simulink model "DCMotorCLDCDC"  (R2018b)
settings: Solver=VariableStepAuto  StartTime=0.0  StopTime=10  RelTol=1e-3  EnableMultiTasking=on
InitFcn:
  | Vf=300;
libraries: powerlib x17, simulink x6, powerlib_meascontrol x2
settings Model: Creator=alireza  LastModifiedBy=Koosha
settings OptimizationCC: LifeSpan=inf
settings DebuggingCC: SFUnexpectedBacktrackingDiag=warning  SFNoUnconditionalDefaultTransitionDiag=warning
settings SFSimCC: SimUseLocalCustomCode=off
settings RTWCC: RTWUseLocalCustomCode=off
settings CodeAppCC: StateflowObjectComments=on
settings GRTTargetCC: TargetLangStandard=C89/C90 (ANSI)
settings ConfigComp: CovMetricSettings=dw  CovSaveCumulativeToWorkspaceVar=on  CovSaveSingleToWorkspaceVar=on  CovExternalEMLEnable=off
settings SimscapeCC: SimscapeNormalizeSystem=off

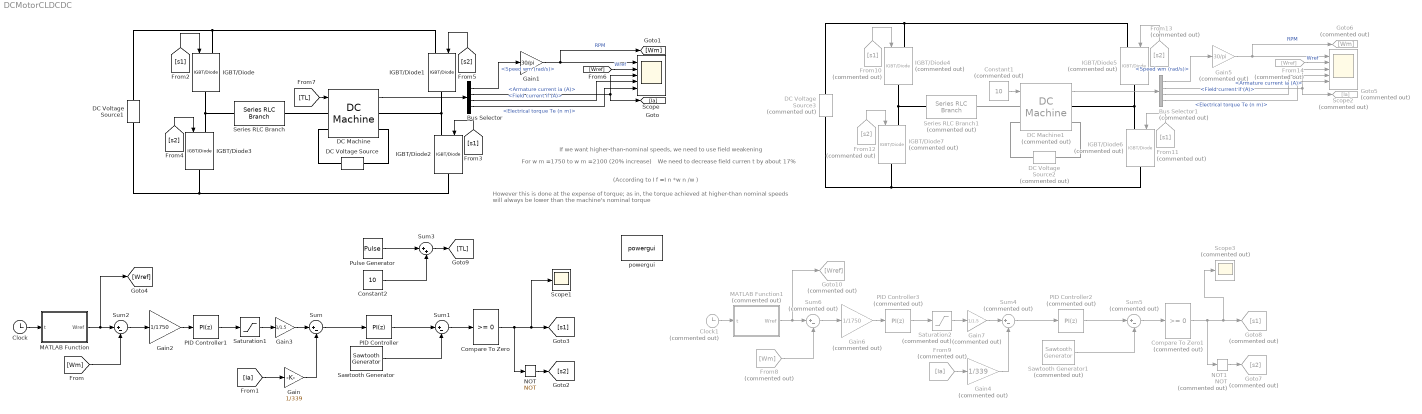
== system DCMotorCLDCDC ==
  note: We need to decrease field curren t by about 17%
  note: However this is done at the expense of torque;
      | as in, the torque achieved at higher-than nominal speeds will always be lower than the machine's nominal torque
  note: For w m =1750 to w m =2100 (20% increase)
  note: (According to I f =I n *w n /w )
  note: If we want higher-than-nominal speeds, we need to use field weakening
  Bus Selector : BusSelector  OutputSignals=Speed wm (rad/s),Armature current ia (A),Field current if (A),Electrical torque Te (n m)
  Bus Selector1 : BusSelector  Commented=on  OutputSignals=Speed wm (rad/s),Armature current ia (A),Field current if (A),Electrical torque Te (n m)
  Clock : Clock
  Clock1 : Clock  Commented=on
  Compare To Zero : simulink/Logic and Bit Operations/Compare To Zero  relop=>=  OutDataTypeStr=boolean
  Compare To Zero1 : simulink/Logic and Bit Operations/Compare To Zero  Commented=on  relop=>=  OutDataTypeStr=boolean
  Constant1 : Constant  Commented=on  Value=10
  Constant2 : Constant  Value=10
  DC Machine : powerlib/Machines/DC Machine  PresetModel=03: 5HP 500V 1750RPM Field:300V  MechanicalLoad=Torque TL  FieldType=Wound  ShowDetailedParameters=on  MeasurementBus=off  RLa=[11.2 0.1215]  RLf=[281.3 156]  Laf=1.976  MachineConstant=Torque constant (N.m/A)  Ke=1.8  Kt=1.8  J=0.02215  Bm=0.002953  Tf=0.5161  w0=0  Ifinit=1  TsPowergui=0  TsBlock=-1
  DC Machine1 : powerlib/Machines/DC Machine  Commented=on  PresetModel=03: 5HP 500V 1750RPM Field:300V  MechanicalLoad=Torque TL  FieldType=Wound  ShowDetailedParameters=on  MeasurementBus=off  RLa=[11.2 0.1215]  RLf=[281.3 156]  Laf=1.976  MachineConstant=Torque constant (N.m/A)  Ke=1.8  Kt=1.8  J=0.02215  Bm=0.002953  Tf=0.5161  w0=0  Ifinit=1  TsPowergui=0  TsBlock=-1
  DC Voltage Source : powerlib/Electrical Sources/DC Voltage Source  Amplitude=300  Measurements=None
  DC Voltage Source1 : powerlib/Electrical Sources/DC Voltage Source  Amplitude=560  Measurements=None
  DC Voltage Source2 : powerlib/Electrical Sources/DC Voltage Source  Commented=on  Amplitude=Vf  Measurements=None
  DC Voltage Source3 : powerlib/Electrical Sources/DC Voltage Source  Commented=on  Amplitude=560  Measurements=None
  From10 : From  Commented=on  GotoTag=s1
  From11 : From  Commented=on  GotoTag=s1
  From12 : From  Commented=on  GotoTag=s2
  From13 : From  Commented=on  GotoTag=s2
  From14 : From  Commented=on  GotoTag=Wref
  From8 : From  Commented=on  GotoTag=Wm
  From9 : From  Commented=on  GotoTag=Ia
  Gain : Gain  Gain=1/339
  Gain1 : Gain  Gain=30/pi
  Gain2 : Gain  Gain=1/1750
  Gain3 : Gain  Gain=1/1.5
  Gain4 : Gain  Commented=on  Gain=1/339
  Gain5 : Gain  Commented=on  Gain=30/pi
  Gain6 : Gain  Commented=on  Gain=1/1750
  Gain7 : Gain  Commented=on  Gain=1/1.5
  Goto10 : Goto  Commented=on  GotoTag=Wref
  Goto5 : Goto  Commented=on  GotoTag=Ia
  Goto6 : Goto  Commented=on  GotoTag=Wm
  Goto7 : Goto  Commented=on  GotoTag=s2
  Goto8 : Goto  Commented=on  GotoTag=s1
  IGBT/Diode{,1..3} (4 alike) : powerlib/Power Electronics/IGBT//Diode  Ron=1e-3  Rs=10e3  Cs=inf  Measurements=off
  IGBT/Diode{4..7} (4 alike) : powerlib/Power Electronics/IGBT//Diode  Commented=on  Ron=1e-3  Rs=10e3  Cs=inf  Measurements=off
  MATLAB Function : MATLAB Function  TreatAsAtomicUnit=on
  MATLAB Function1 : MATLAB Function  Commented=on  TreatAsAtomicUnit=on
  NOT : Logic  Operator=NOT  IconShape=distinctive  AllPortsSameDT=off  OutDataTypeStr=boolean
  NOT1 : Logic  Commented=on  Operator=NOT  IconShape=distinctive  AllPortsSameDT=off  OutDataTypeStr=boolean
  PID Controller : simulink/Continuous/PID Controller  Controller=PI  Form=Parallel  TimeDomain=Discrete-time  SampleTime=-1  IntegratorMethod=Forward Euler  FilterMethod=Forward Euler  ControllerParametersSource=internal  P=5  I=6  D=0  UseFilter=on  N=100  TunerSelectOption=Transfer Function Based (PID Tuner App)  InitialConditionSource=internal  InitialConditionForIntegrator=0  InitialConditionForFilter=0  DifferentiatorICPrevScaledInput=0  ExternalReset=none  TrackingMode=off  Kt=1  LimitOutput=off  UpperSaturationLimit=inf  LowerSaturationLimit=-inf  LinearizeAsGain=on  AntiWindupMode=none  Kb=1  POutMin=[]  POutMax=[]  IOutMin=[]  IOutMax=[]  DOutMin=[]  DOutMax=[]  NOutMin=[]  NOutMax=[]  SumOutMin=[]  SumOutMax=[]  SaturationOutMin=[]  SaturationOutMax=[]  PParamMin=[]  PParamMax=[]  IParamMin=[]  IParamMax=[]  DParamMin=[]  DParamMax=[]  NParamMin=[]  NParamMax=[]  KbParamMin=[]  KbParamMax=[]  KtParamMin=[]  KtParamMax=[]  KbOutMin=[]  KbOutMax=[]  KtOutMin=[]  KtOutMax=[]  IntegratorOutMin=[]  IntegratorOutMax=[]  FilterOutMin=[]  FilterOutMax=[]  SumI1OutMin=[]  SumI1OutMax=[]  SumI2OutMin=[]  SumI2OutMax=[]  SumI3OutMin=[]  SumI3OutMax=[]  SumI4OutMin=[]  SumI4OutMax=[]  SumDOutMin=[]  SumDOutMax=[]  DifferentiatorOutMin=[]  DifferentiatorOutMax=[]  FilterDiffOutCoefMin=[]  FilterDiffOutCoefMax=[]  ReciprocalOutMin=[]  ReciprocalOutMax=[]  SumDenOutMin=[]  SumDenOutMax=[]  SumNumOutMin=[]  SumNumOutMax=[]  DivideOutMin=[]  DivideOutMax=[]  IntegratorContinuousStateAttributes=''  IntegratorStateMustResolveToSignalObject=off  IntegratorRTWStateStorageClass=Auto  FilterContinuousStateAttributes=''  FilterStateMustResolveToSignalObject=off  FilterRTWStateStorageClass=Auto  ParallelPVariant=InternalParameters  IdealPVariant=Disabled  IVariant=InternalParameters  DVariant=Disabled  IntegratorVariant=Discrete  SatVariant=Disabled  AWVariant=Passthrough  PCopyVariant=Disabled  TRVariant=Disabled  FdbkBlocksVariant=Forward  IdealPFdbkVariant=Disabled  SatFdbkVariant=Disabled  DerivativeFilterVariant=Disabled  NVariant=Disabled  NCopyVariant=Disabled_SignalSpec  FilterICVariant=Disabled  IntegratorICVariant=InternalICs  ExternalResetVariant=Disabled  TRSumVariant=Passthrough  SumFdbkVariant=Disabled  SumVariant=Sum_PI
  PID Controller1 : simulink/Continuous/PID Controller  Controller=PI  Form=Parallel  TimeDomain=Discrete-time  SampleTime=-1  IntegratorMethod=Forward Euler  FilterMethod=Forward Euler  ControllerParametersSource=internal  P=10  I=10  D=0  UseFilter=on  N=100  TunerSelectOption=Transfer Function Based (PID Tuner App)  InitialConditionSource=internal  InitialConditionForIntegrator=0  InitialConditionForFilter=0  DifferentiatorICPrevScaledInput=0  ExternalReset=none  TrackingMode=off  Kt=1  LimitOutput=off  UpperSaturationLimit=inf  LowerSaturationLimit=-inf  LinearizeAsGain=on  AntiWindupMode=none  Kb=1  POutMin=[]  POutMax=[]  IOutMin=[]  IOutMax=[]  DOutMin=[]  DOutMax=[]  NOutMin=[]  NOutMax=[]  SumOutMin=[]  SumOutMax=[]  SaturationOutMin=[]  SaturationOutMax=[]  PParamMin=[]  PParamMax=[]  IParamMin=[]  IParamMax=[]  DParamMin=[]  DParamMax=[]  NParamMin=[]  NParamMax=[]  KbParamMin=[]  KbParamMax=[]  KtParamMin=[]  KtParamMax=[]  KbOutMin=[]  KbOutMax=[]  KtOutMin=[]  KtOutMax=[]  IntegratorOutMin=[]  IntegratorOutMax=[]  FilterOutMin=[]  FilterOutMax=[]  SumI1OutMin=[]  SumI1OutMax=[]  SumI2OutMin=[]  SumI2OutMax=[]  SumI3OutMin=[]  SumI3OutMax=[]  SumI4OutMin=[]  SumI4OutMax=[]  SumDOutMin=[]  SumDOutMax=[]  DifferentiatorOutMin=[]  DifferentiatorOutMax=[]  FilterDiffOutCoefMin=[]  FilterDiffOutCoefMax=[]  ReciprocalOutMin=[]  ReciprocalOutMax=[]  SumDenOutMin=[]  SumDenOutMax=[]  SumNumOutMin=[]  SumNumOutMax=[]  DivideOutMin=[]  DivideOutMax=[]  IntegratorContinuousStateAttributes=''  IntegratorStateMustResolveToSignalObject=off  IntegratorRTWStateStorageClass=Auto  FilterContinuousStateAttributes=''  FilterStateMustResolveToSignalObject=off  FilterRTWStateStorageClass=Auto  ParallelPVariant=InternalParameters  IdealPVariant=Disabled  IVariant=InternalParameters  DVariant=Disabled  IntegratorVariant=Discrete  SatVariant=Disabled  AWVariant=Passthrough  PCopyVariant=Disabled  TRVariant=Disabled  FdbkBlocksVariant=Forward  IdealPFdbkVariant=Disabled  SatFdbkVariant=Disabled  DerivativeFilterVariant=Disabled  NVariant=Disabled  NCopyVariant=Disabled_SignalSpec  FilterICVariant=Disabled  IntegratorICVariant=InternalICs  ExternalResetVariant=Disabled  TRSumVariant=Passthrough  SumFdbkVariant=Disabled  SumVariant=Sum_PI
  PID Controller2 : simulink/Continuous/PID Controller  Commented=on  Controller=PI  Form=Parallel  TimeDomain=Discrete-time  SampleTime=-1  IntegratorMethod=Forward Euler  FilterMethod=Forward Euler  ControllerParametersSource=internal  P=5  I=6  D=0  UseFilter=on  N=100  TunerSelectOption=Transfer Function Based (PID Tuner App)  InitialConditionSource=internal  InitialConditionForIntegrator=0  InitialConditionForFilter=0  DifferentiatorICPrevScaledInput=0  ExternalReset=none  TrackingMode=off  Kt=1  LimitOutput=off  UpperSaturationLimit=inf  LowerSaturationLimit=-inf  LinearizeAsGain=on  AntiWindupMode=none  Kb=1  POutMin=[]  POutMax=[]  IOutMin=[]  IOutMax=[]  DOutMin=[]  DOutMax=[]  NOutMin=[]  NOutMax=[]  SumOutMin=[]  SumOutMax=[]  SaturationOutMin=[]  SaturationOutMax=[]  PParamMin=[]  PParamMax=[]  IParamMin=[]  IParamMax=[]  DParamMin=[]  DParamMax=[]  NParamMin=[]  NParamMax=[]  KbParamMin=[]  KbParamMax=[]  KtParamMin=[]  KtParamMax=[]  KbOutMin=[]  KbOutMax=[]  KtOutMin=[]  KtOutMax=[]  IntegratorOutMin=[]  IntegratorOutMax=[]  FilterOutMin=[]  FilterOutMax=[]  SumI1OutMin=[]  SumI1OutMax=[]  SumI2OutMin=[]  SumI2OutMax=[]  SumI3OutMin=[]  SumI3OutMax=[]  SumI4OutMin=[]  SumI4OutMax=[]  SumDOutMin=[]  SumDOutMax=[]  DifferentiatorOutMin=[]  DifferentiatorOutMax=[]  FilterDiffOutCoefMin=[]  FilterDiffOutCoefMax=[]  ReciprocalOutMin=[]  ReciprocalOutMax=[]  SumDenOutMin=[]  SumDenOutMax=[]  SumNumOutMin=[]  SumNumOutMax=[]  DivideOutMin=[]  DivideOutMax=[]  IntegratorContinuousStateAttributes=''  IntegratorStateMustResolveToSignalObject=off  IntegratorRTWStateStorageClass=Auto  FilterContinuousStateAttributes=''  FilterStateMustResolveToSignalObject=off  FilterRTWStateStorageClass=Auto  ParallelPVariant=InternalParameters  IdealPVariant=Disabled  IVariant=InternalParameters  DVariant=Disabled  IntegratorVariant=Discrete  SatVariant=Disabled  AWVariant=Passthrough  PCopyVariant=Disabled  TRVariant=Disabled  FdbkBlocksVariant=Forward  IdealPFdbkVariant=Disabled  SatFdbkVariant=Disabled  DerivativeFilterVariant=Disabled  NVariant=Disabled  NCopyVariant=Disabled_SignalSpec  FilterICVariant=Disabled  IntegratorICVariant=InternalICs  ExternalResetVariant=Disabled  TRSumVariant=Passthrough  SumFdbkVariant=Disabled  SumVariant=Sum_PI
  PID Controller3 : simulink/Continuous/PID Controller  Commented=on  Controller=PI  Form=Parallel  TimeDomain=Discrete-time  SampleTime=-1  IntegratorMethod=Forward Euler  FilterMethod=Forward Euler  ControllerParametersSource=internal  P=10  I=10  D=0  UseFilter=on  N=100  TunerSelectOption=Transfer Function Based (PID Tuner App)  InitialConditionSource=internal  InitialConditionForIntegrator=0  InitialConditionForFilter=0  DifferentiatorICPrevScaledInput=0  ExternalReset=none  TrackingMode=off  Kt=1  LimitOutput=off  UpperSaturationLimit=inf  LowerSaturationLimit=-inf  LinearizeAsGain=on  AntiWindupMode=none  Kb=1  POutMin=[]  POutMax=[]  IOutMin=[]  IOutMax=[]  DOutMin=[]  DOutMax=[]  NOutMin=[]  NOutMax=[]  SumOutMin=[]  SumOutMax=[]  SaturationOutMin=[]  SaturationOutMax=[]  PParamMin=[]  PParamMax=[]  IParamMin=[]  IParamMax=[]  DParamMin=[]  DParamMax=[]  NParamMin=[]  NParamMax=[]  KbParamMin=[]  KbParamMax=[]  KtParamMin=[]  KtParamMax=[]  KbOutMin=[]  KbOutMax=[]  KtOutMin=[]  KtOutMax=[]  IntegratorOutMin=[]  IntegratorOutMax=[]  FilterOutMin=[]  FilterOutMax=[]  SumI1OutMin=[]  SumI1OutMax=[]  SumI2OutMin=[]  SumI2OutMax=[]  SumI3OutMin=[]  SumI3OutMax=[]  SumI4OutMin=[]  SumI4OutMax=[]  SumDOutMin=[]  SumDOutMax=[]  DifferentiatorOutMin=[]  DifferentiatorOutMax=[]  FilterDiffOutCoefMin=[]  FilterDiffOutCoefMax=[]  ReciprocalOutMin=[]  ReciprocalOutMax=[]  SumDenOutMin=[]  SumDenOutMax=[]  SumNumOutMin=[]  SumNumOutMax=[]  DivideOutMin=[]  DivideOutMax=[]  IntegratorContinuousStateAttributes=''  IntegratorStateMustResolveToSignalObject=off  IntegratorRTWStateStorageClass=Auto  FilterContinuousStateAttributes=''  FilterStateMustResolveToSignalObject=off  FilterRTWStateStorageClass=Auto  ParallelPVariant=InternalParameters  IdealPVariant=Disabled  IVariant=InternalParameters  DVariant=Disabled  IntegratorVariant=Discrete  SatVariant=Disabled  AWVariant=Passthrough  PCopyVariant=Disabled  TRVariant=Disabled  FdbkBlocksVariant=Forward  IdealPFdbkVariant=Disabled  SatFdbkVariant=Disabled  DerivativeFilterVariant=Disabled  NVariant=Disabled  NCopyVariant=Disabled_SignalSpec  FilterICVariant=Disabled  IntegratorICVariant=InternalICs  ExternalResetVariant=Disabled  TRSumVariant=Passthrough  SumFdbkVariant=Disabled  SumVariant=Sum_PI
  Pulse Generator : DiscretePulseGenerator  PulseType=Time based  Amplitude=10  Period=10  PulseWidth=40  PhaseDelay=4
  Saturation1 : Saturate  UpperLimit=1.5  LowerLimit=-1.5
  Saturation2 : Saturate  Commented=on  UpperLimit=1.5  LowerLimit=-1.5
  Sawtooth Generator : powerlib_meascontrol/Pulse & Signal Generators/Sawtooth Generator  Freq=5e3  Phase=90  Ts=20e-6
      settings: SourceProductName=Simscape Power Systems
  Sawtooth Generator1 : powerlib_meascontrol/Pulse & Signal Generators/Sawtooth Generator  Commented=on  Freq=5e3  Phase=90  Ts=20e-6
      settings: SourceProductName=Simscape Power Systems
  Scope : Scope  NumInputPorts=5
  Scope1 : Scope
  Scope2 : Scope  Commented=on  NumInputPorts=5
  Scope3 : Scope  Commented=on
  Series RLC Branch : powerlib/Elements/Series RLC Branch  LConnTagsString=__new0  RConnTagsString=__new0  BranchType=L  Resistance=1  Inductance=1e-3  SetiL0=off  InitialCurrent=0  Capacitance=1e-6  Setx0=off  InitialVoltage=0  Measurements=None
  Series RLC Branch1 : powerlib/Elements/Series RLC Branch  Commented=on  LConnTagsString=__new0  RConnTagsString=__new0  BranchType=L  Resistance=1  Inductance=1e-3  SetiL0=off  InitialCurrent=0  Capacitance=1e-6  Setx0=off  InitialVoltage=0  Measurements=None
  Sum : Sum  Inputs=|+-
  Sum1 : Sum  Inputs=|+-
  Sum2 : Sum  Inputs=|+-
  Sum3 : Sum  Inputs=|++
  Sum4 : Sum  Commented=on  Inputs=|+-
  Sum5 : Sum  Commented=on  Inputs=|+-
  Sum6 : Sum  Commented=on  Inputs=|+-
  powergui : powerlib/powergui  Priority=1  SimulationMode=Discrete  SampleTime=50e-6  frequency=60  Iterations=50  frequencyindice=0  Pbase=100e6  ErrMax=1e-4  UnitsV=kV  UnitsW=MW  buscounter=0  FunctionMessages=off  echomessages=off  EnableUseOfTLC=off  CurrentSourceSwitches=off  DisableSnubberDevices=off  DisableRonSwitches=off  DisableVfSwitches=off  DisplayEquations=off  SolverType=Tustin/Backward Euler (TBE)  Interpol=off  ExternalGateDelay=off  methode=off  Ts=100  x0status=blocks  SPID=off  SwTol=0  HookPort=off  RestoreLinks=warning  ResistiveCurrentMeasurement=off  Frange=[0:2:500]  Ylog=off  Xlog=on  ShowGrid=off  save=off  variable=ZData  structure=0  ZoomFFT=off  StartTime=0.0  cycles=1  DisplayStyle=1  fundamental=60  FreqAxis=off  MaxFrequency=1000  frequencyindicesteady=1  RmsSteady=1  display=off
  wires:
  Sum/1 -> PID Controller/1
  Sawtooth Generator/1 -> Sum1/2
  Sum1/1 -> Compare To Zero/1
  Clock/1 -> MATLAB Function/1(t)
  DC Machine/1 -> Bus Selector/1
  Bus Selector/1 -> Gain1/1  "<Speed wm (rad/s)>"
  MATLAB Function/1(Wref) -> [Wref], Sum2/1
  [Wm] -> Sum2/2
  Gain1/1 -> [Wm], Scope/1  "RPM"
  PID Controller1/1 -> Saturation1/1
  Compare To Zero/1 -> NOT/1, Scope1/1, [s1]
  NOT/1 -> [s2]
  [s1] -> IGBT/Diode/1
  [s1] -> IGBT/Diode2/1
  [s2] -> IGBT/Diode3/1
  [s2] -> IGBT/Diode1/1
  PID Controller/1 -> Sum1/1
  [Wref] -> Scope/2  "Wref"
  Bus Selector/2 -> [Ia], Scope/3  "<Armature current ia (A)>"
  Bus Selector/4 -> Scope/5  "<Electrical torque Te (n m)>"
  Bus Selector/3 -> Scope/4  "<Field current if (A)>"
  Saturation1/1 -> Gain3/1
  [Ia] -> Gain/1
  Gain/1 -> Sum/2
  Gain3/1 -> Sum/1
  Gain2/1 -> PID Controller1/1
  Sum2/1 -> Gain2/1
  Constant2/1 -> Sum3/2
  Sum3/1 -> [TL]
  Pulse Generator/1 -> Sum3/1
  [TL] -> DC Machine/1
  Constant1/1 -> DC Machine1/1
  Gain5/1 -> Goto6/1, Scope2/1  "RPM"
  Sum6/1 -> Gain6/1
  Gain7/1 -> Sum4/1
  Bus Selector1/4 -> Scope2/5  "<Electrical torque Te (n m)>"
  Sawtooth Generator1/1 -> Sum5/2
  PID Controller2/1 -> Sum5/1
  Gain6/1 -> PID Controller3/1
  Bus Selector1/1 -> Gain5/1  "<Speed wm (rad/s)>"
  From10/1 -> IGBT/Diode4/1
  DC Machine1/1 -> Bus Selector1/1
  From12/1 -> IGBT/Diode7/1
  From13/1 -> IGBT/Diode5/1
  From11/1 -> IGBT/Diode6/1
  NOT1/1 -> Goto7/1
  MATLAB Function1/1(Wref) -> Goto10/1, Sum6/1
  Bus Selector1/3 -> Scope2/4  "<Field current if (A)>"
  Saturation2/1 -> Gain7/1
  Bus Selector1/2 -> Goto5/1, Scope2/3  "<Armature current ia (A)>"
  Clock1/1 -> MATLAB Function1/1(t)
  From14/1 -> Scope2/2  "Wref"
  Sum4/1 -> PID Controller2/1
  Compare To Zero1/1 -> NOT1/1, Scope3/1, Goto8/1
  Sum5/1 -> Compare To Zero1/1
  PID Controller3/1 -> Saturation2/1
  From8/1 -> Sum6/2
  From9/1 -> Gain4/1
  Gain4/1 -> Sum4/2
  connections:
  IGBT/Diode1/RConn1 -- DC Machine/RConn1 -- IGBT/Diode2/LConn1
  DC Voltage Source/RConn1 -- DC Machine/LConn2
  DC Voltage Source/LConn1 -- DC Machine/RConn2
  DC Machine/LConn1 -- Series RLC Branch/RConn1
  IGBT/Diode3/LConn1 -- Series RLC Branch/LConn1 -- IGBT/Diode/RConn1
  IGBT/Diode/LConn1 -- DC Voltage Source1/RConn1 -- IGBT/Diode1/LConn1
  IGBT/Diode2/RConn1 -- DC Voltage Source1/LConn1 -- IGBT/Diode3/RConn1
  IGBT/Diode4/RConn1 -- IGBT/Diode7/LConn1 -- Series RLC Branch1/LConn1
  IGBT/Diode5/LConn1 -- IGBT/Diode4/LConn1 -- DC Voltage Source3/RConn1
  IGBT/Diode7/RConn1 -- IGBT/Diode6/RConn1 -- DC Voltage Source3/LConn1
  IGBT/Diode6/LConn1 -- IGBT/Diode5/RConn1 -- DC Machine1/RConn1
  DC Voltage Source2/RConn1 -- DC Machine1/LConn2
  DC Machine1/LConn1 -- Series RLC Branch1/RConn1
  DC Voltage Source2/LConn1 -- DC Machine1/RConn2

== matlab function DCMotorCLDCDC/MATLAB Function1 ==
  data: t input; Wref output

function Wref = fcn(t)

W = 1750;   

if t < 1
    Wref = 0;

elseif t < 3    
    Wref = W;

elseif t < 5 
    Vf = 270;
    Wref = 1.2*W;

elseif t < 7
    Vf = 300;
    Wref = -W;

elseif t < 9
    Vf = 270;
    Wref = -1.2*W;

else
    Vf = 300;
    Wref = 0;

end

== matlab function DCMotorCLDCDC/MATLAB Function ==
  data: t input; Wref output

function Wref = fcn(t)

W = 1750;   

if t < 1
    Wref = 0;

elseif t < 3    
    Wref = 0.5*W;

elseif t < 5 
    Wref = W;

elseif t < 7
    Wref = -0.5*W;

elseif t < 9
    Wref = -W;

else
    Wref = 0;

end
